simulink model "ideal_model"  (R2015b)
settings: Solver=VariableStepAuto  StartTime=0.0  StopTime=10.0  RelTol=1e-3
settings Model: Creator=yuji  LastModifiedBy=yuji

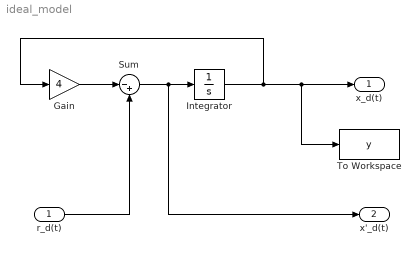
== system ideal_model ==
  r_d(t) : Inport
  Gain : Gain  Gain=4
  Integrator : Integrator
  Sum : Sum  Inputs=|-+
  To Workspace : ToWorkspace  VariableName=y  SaveFormat=Timeseries  SampleTime=-1
  x_d(t) : Outport
  x'_d(t) : Outport  Port=2
  wires:
  Integrator/1 -> Gain/1, To Workspace/1, x_d(t)/1
  Sum/1 -> x'_d(t)/1, Integrator/1
  r_d(t)/1 -> Sum/2
  Gain/1 -> Sum/1
